simulink model "tentando_arrumar_encoder"  (R2012b)
settings: Solver=ode45  StartTime=0.0  StopTime=2  MaxStep=1e-4  RelTol=1e-3
libraries: simulink x4, Encoder x1
settings Model: Creator=Juliano  LastModifiedBy=Juliano

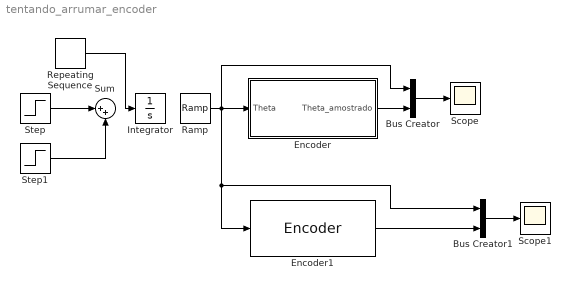
== system tentando_arrumar_encoder ==
  Bus Creator : BusCreator  Inputs=2
  Bus Creator1 : BusCreator  Inputs=2
  Encoder : Subsystem  AncestorBlock=Encoder/Encoder  mask(Encoder de quadratura){Nr=50}
      mask prompts: Nr "Número de pulsos por revolução"
      mask help:
      | Simula o funcionamento de um encoder de quadratura.
      |
      | Entradas
      | - Theta: ângulo real [graus]
      | Saídas
      | - Theta_amostrado: ângulo que um encoder mostraria [graus]
  Encoder1 : Encoder/Encoder  Nr=50
  Integrator : Integrator
  Ramp : simulink/Sources/Ramp  slope=-36  start=0  X0=0
  Repeating Sequence : simulink/Sources/Repeating Sequence  rep_seq_t=[0 1]  rep_seq_y=[36 -50]
  Scope : Scope
  Scope1 : Scope
      settings: SaveName=ScopeData2
  Step : Step  Time=0  After=36  SampleTime=0
  Step1 : Step  After=-72  SampleTime=0
  Sum : Sum  Inputs=|++
  wires:
  Encoder/1(Theta_amostrado) -> Bus Creator/2
  Bus Creator/1 -> Scope/1
  Ramp/1 -> Bus Creator/1, Encoder1/1, Bus Creator1/1, Encoder/1(Theta)
  Encoder1/1 -> Bus Creator1/2
  Bus Creator1/1 -> Scope1/1
  Step/1 -> Sum/1
  Step1/1 -> Sum/2
  Repeating Sequence/1 -> Integrator/1

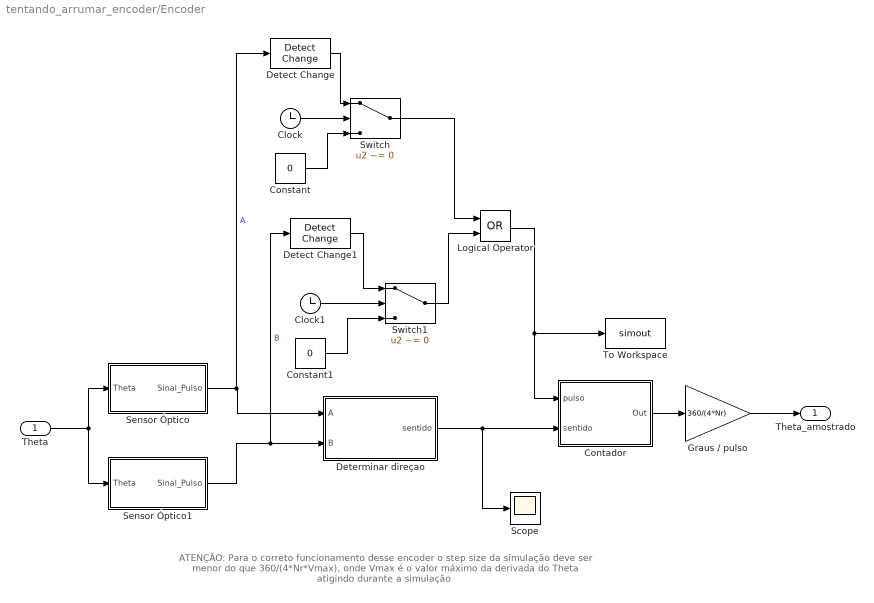
== system tentando_arrumar_encoder/Encoder ==
  note: ATENÇÃO: Para o correto funcionamento desse encoder o step size da simulação deve ser menor do que 360/(4*Nr*Vmax),
      | onde Vmax é o valor máximo da derivada do Theta atigindo durante a simulação
  Theta : Inport
  Clock : Clock
  Clock1 : Clock
  Constant : Constant  Value=0
  Constant1 : Constant  Value=0
  Contador : Subsystem
  Detect Change : simulink/Logic and Bit Operations/Detect Change  vinit=0  InputProcessing=Inherited  OutDataTypeStr=uint8
  Detect Change1 : simulink/Logic and Bit Operations/Detect Change  vinit=0  InputProcessing=Inherited  OutDataTypeStr=uint8
  Determinar direçao : Subsystem
  Graus / pulso : Gain  Gain=360/(4*Nr)  OutDataTypeStr=double
  Logical Operator : Logic  Operator=OR  AllPortsSameDT=off  OutDataTypeStr=boolean
  Scope : Scope
  Sensor Óptico : Subsystem
  Sensor Óptico1 : Subsystem
  Switch : Switch  Criteria=u2 ~= 0
  Switch1 : Switch  Criteria=u2 ~= 0
  To Workspace : ToWorkspace  VariableName=simout  SampleTime=-1  SaveFormat=Timeseries
  Theta_amostrado : Outport
  wires:
  Theta/1 -> Sensor Óptico/1(Theta), Sensor Óptico1/1(Theta)
  Graus / pulso/1 -> Theta_amostrado/1
  Contador/1(Out) -> Graus / pulso/1
  Sensor Óptico1/1(Sinal_Pulso) -> Detect Change1/1, Determinar direçao/2(B)  "B"
  Sensor Óptico/1(Sinal_Pulso) -> Detect Change/1, Determinar direçao/1(A)  "A"
  Determinar direçao/1(sentido) -> Scope/1, Contador/2(sentido)
  Switch/1 -> Logical Operator/1
  Logical Operator/1 -> To Workspace/1, Contador/1(pulso)
  Switch1/1 -> Logical Operator/2
  Clock/1 -> Switch/2
  Constant/1 -> Switch/3
  Detect Change/1 -> Switch/1
  Clock1/1 -> Switch1/2
  Constant1/1 -> Switch1/3
  Detect Change1/1 -> Switch1/1

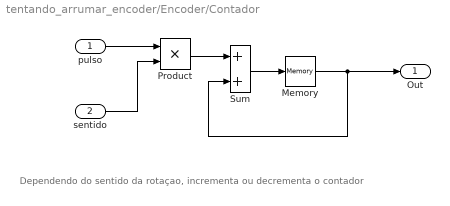
== system tentando_arrumar_encoder/Encoder/Contador ==
  note: Dependendo do sentido da rotaçao, incrementa ou decrementa o contador
  pulso : Inport
  sentido : Inport  Port=2
  Memory : Memory
  Product : Product  RndMeth=Zero
  Sum : Sum
  Out : Outport
  wires:
  Sum/1 -> Memory/1
  Memory/1 -> Out/1, Sum/2
  pulso/1 -> Product/1
  sentido/1 -> Product/2
  Product/1 -> Sum/1

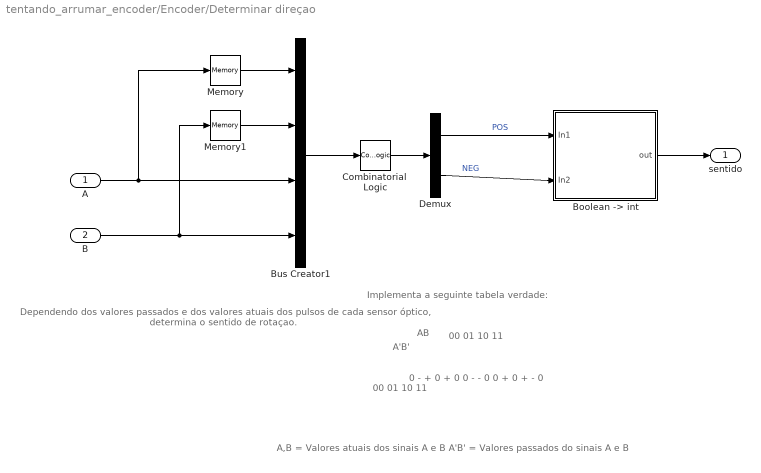
== system tentando_arrumar_encoder/Encoder/Determinar direçao ==
  note: Dependendo dos valores passados e dos valores atuais
      | dos pulsos de cada sensor óptico, determina o sentido
      | de rotaçao.
  note: 00
      | 01
      | 10
      | 11
  note: 00 01 10 11
  note: 0	-	+	0
      | +	0	0	-
      | -	0	0	+
      | 0	+	-	0
  note: Implementa a seguinte tabela verdade:
  note: AB
  note: A'B'
  note: A,B = Valores atuais dos sinais A e B
      | A'B' = Valores passados do sinais A e B
  A : Inport
  B : Inport  Port=2
  "Boolean -> int " : Subsystem
  Bus Creator1 : BusCreator
  Combinatorial  Logic : CombinatorialLogic  TruthTable=[ 0 0 ; 0 1 ; 1 0 ; 0 0 ; 1 0 ; 0 0 ; 0 0 ; 0 1 ; 0 1 ; 0 0 ; 0 0 ; 1 0 ; 0 0 ; 1 0 ; 0 1 ; 0 0]
  Demux : Demux  Outputs=2
  Memory : Memory
  Memory1 : Memory
  sentido : Outport
  wires:
  B/1 -> Bus Creator1/4, Memory1/1
  Memory1/1 -> Bus Creator1/2
  Bus Creator1/1 -> Combinatorial  Logic/1
  Memory/1 -> Bus Creator1/1
  Combinatorial  Logic/1 -> Demux/1
  A/1 -> Bus Creator1/3, Memory/1
  Demux/1 -> "Boolean -> int "/1(In1)  "POS"
  Demux/2 -> "Boolean -> int "/2(In2)  "NEG"
  "Boolean -> int "/1(out) -> sentido/1

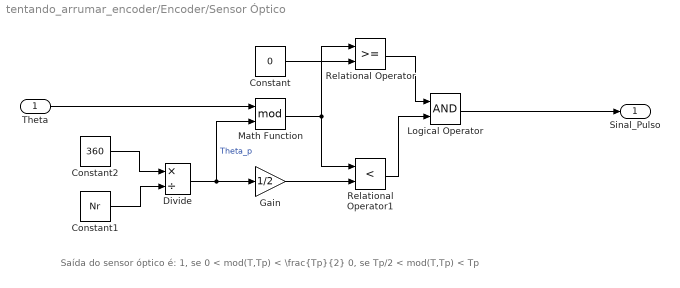
== system tentando_arrumar_encoder/Encoder/Sensor Óptico ==
  note: Saída do sensor óptico é:
      | 1, se	0 < mod(T,Tp) < \frac{Tp}{2}
      |  0, se      Tp/2 < mod(T,Tp) < Tp
  Theta : Inport
  Constant : Constant  Value=0
  Constant1 : Constant  Value=Nr
  Constant2 : Constant  Value=360
  Divide : Product  Inputs=*/
  Gain : Gain  Gain=1/2
  Logical Operator : Logic  AllPortsSameDT=off  OutDataTypeStr=boolean
  Math Function : Math  Operator=mod  SaturateOnIntegerOverflow=on
  Relational Operator : RelationalOperator  OutDataTypeStr=boolean
  Relational Operator1 : RelationalOperator  Operator=<  OutDataTypeStr=boolean
  Sinal_Pulso : Outport
  wires:
  Constant1/1 -> Divide/2
  Constant2/1 -> Divide/1
  Gain/1 -> Relational Operator1/2
  Divide/1 -> Gain/1, Math Function/2  "Theta_p"
  Constant/1 -> Relational Operator/2
  Relational Operator1/1 -> Logical Operator/2
  Relational Operator/1 -> Logical Operator/1
  Theta/1 -> Math Function/1
  Math Function/1 -> Relational Operator/1, Relational Operator1/1
  Logical Operator/1 -> Sinal_Pulso/1

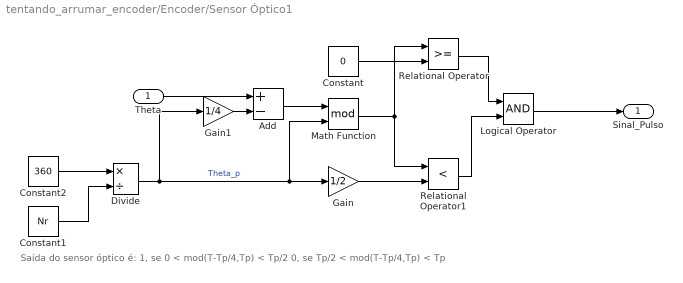
== system tentando_arrumar_encoder/Encoder/Sensor Óptico1 ==
  note: Saída do sensor óptico é:
      | 1, se	0 < mod(T-Tp/4,Tp) < Tp/2
      |  0, se     Tp/2 < mod(T-Tp/4,Tp) < Tp
  Theta : Inport
  Add : Sum  Inputs=+-
  Constant : Constant  Value=0
  Constant1 : Constant  Value=Nr
  Constant2 : Constant  Value=360
  Divide : Product  Inputs=*/
  Gain : Gain  Gain=1/2
  Gain1 : Gain  Gain=1/4
  Logical Operator : Logic  AllPortsSameDT=off  OutDataTypeStr=boolean
  Math Function : Math  Operator=mod  SaturateOnIntegerOverflow=on
  Relational Operator : RelationalOperator  OutDataTypeStr=boolean
  Relational Operator1 : RelationalOperator  Operator=<  OutDataTypeStr=boolean
  Sinal_Pulso : Outport
  wires:
  Gain1/1 -> Add/2
  Theta/1 -> Add/1
  Add/1 -> Math Function/1
  Math Function/1 -> Relational Operator1/1, Relational Operator/1
  Relational Operator/1 -> Logical Operator/1
  Relational Operator1/1 -> Logical Operator/2
  Constant/1 -> Relational Operator/2
  Divide/1 -> Math Function/2, Gain/1, Gain1/1  "Theta_p"
  Gain/1 -> Relational Operator1/2
  Logical Operator/1 -> Sinal_Pulso/1
  Constant2/1 -> Divide/1
  Constant1/1 -> Divide/2

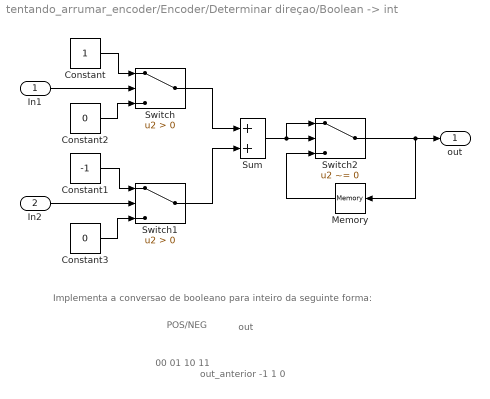
== system tentando_arrumar_encoder/Encoder/Determinar direçao/Boolean -> int  ==
  note: Implementa a conversao de booleano para inteiro da seguinte forma:
  note: out_anterior
      | -1
      | 1
      | 0
  note: 00
      | 01
      | 10
      | 11
  note: out
  note: POS/NEG
  In1 : Inport
  In2 : Inport  Port=2
  Constant : Constant
  Constant1 : Constant  Value=-1
  Constant2 : Constant  Value=0
  Constant3 : Constant  Value=0
  Memory : Memory
  Sum : Sum
  Switch : Switch  Criteria=u2 > Threshold
  Switch1 : Switch  Criteria=u2 > Threshold
  Switch2 : Switch  Criteria=u2 ~= 0
  out : Outport
  wires:
  In1/1 -> Switch/2
  Constant/1 -> Switch/1
  In2/1 -> Switch1/2
  Constant1/1 -> Switch1/1
  Constant3/1 -> Switch1/3
  Constant2/1 -> Switch/3
  Switch/1 -> Sum/1
  Switch1/1 -> Sum/2
  Sum/1 -> Switch2/1, Switch2/2
  Memory/1 -> Switch2/3
  Switch2/1 -> Memory/1, out/1
